simulink model "smartHome6"  (Simulink 9.1)
settings: Solver=VariableStepAuto  StartTime=0.0  StopTime=100  RelTol=1e-3
libraries: commrandsrc3 x21, simulink x8
settings Model: Creator=afarooq  LastModifiedBy=afarooq
settings DataIOCC: SaveFormat=Dataset
settings OptimizationCC: LifeSpan=auto
settings DebuggingCC: UnderspecifiedInitializationDetection=Simplified  MergeDetectMultiDrivingBlocksExec=error  SFUnexpectedBacktrackingDiag=error  SFNoUnconditionalDefaultTransitionDiag=error  SFExecutionAtInitializationDiag=warning
settings HardwareCC: ProdBitPerPointer=64  ProdBitPerSizeT=64  ProdBitPerPtrDiffT=64  ProdLargestAtomicFloat=Float  ProdIntDivRoundTo=Zero  ProdEndianess=LittleEndian  ProdWordSize=64  ProdHWDeviceType=Intel->x86-64 (Windows64)
settings ModelReferenceCC: PropagateSignalLabelsOutOfModel=on
settings CodeAppCC: StateflowObjectComments=off
settings GRTTargetCC: TargetLangStandard=C99 (ISO)  CombineOutputUpdateFcns=on  GRTInterface=off
settings ConfigComp: CovMetricSettings=dwe  CovHtmlReporting=off  CovSaveCumulativeToWorkspaceVar=off  CovSaveSingleToWorkspaceVar=off  CovExternalEMLEnable=on

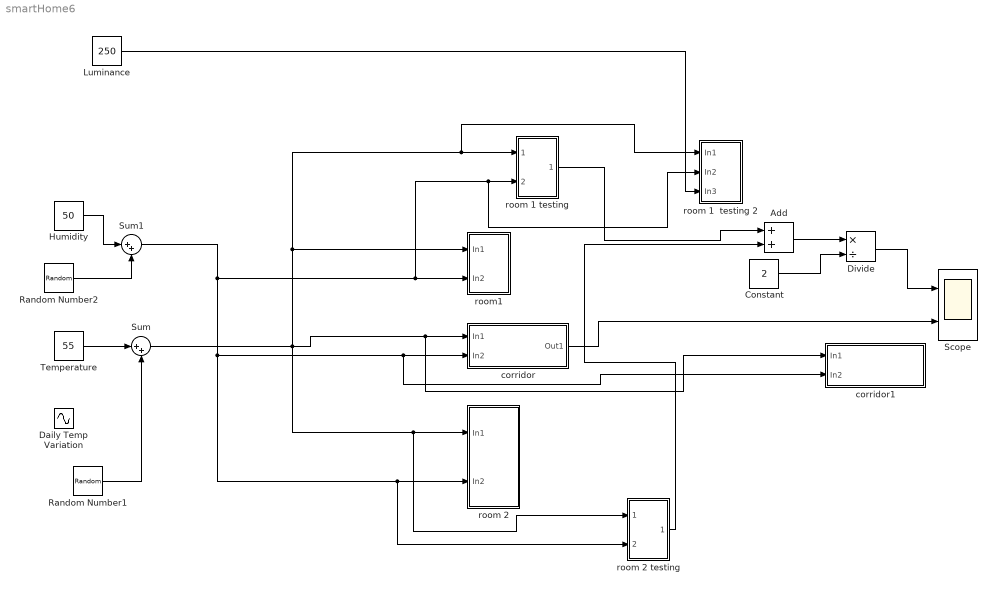
== system smartHome6 ==
  Add : Sum
  Constant : Constant  Value=2
  Daily Temp Variation : Sin  Amplitude=10  Frequency=2*pi/24  SampleTime=0
  Divide : Product  Inputs=*/
  Humidity : Constant  Value=50
  Luminance : Constant  Value=250
  Random Number1 : RandomNumber  Mean=10  Variance=15  SampleTime=1.0
  Random Number2 : RandomNumber  Mean=10  Variance=15  SampleTime=1.0
  Scope : Scope  NumInputPorts=2
  Sum : Sum  Inputs=|++
  Sum1 : Sum  Inputs=|++
  Temperature : Constant  Value=55
  corridor : Subsystem
  corridor1 : Subsystem
  room 1  testing 2 : Subsystem
  "room 1 testing " : Subsystem
  room 2 : Subsystem
  "room 2 testing " : Subsystem
  room1 : Subsystem
  wires:
  Temperature/1 -> Sum/1
  Humidity/1 -> Sum1/1
  Random Number2/1 -> Sum1/2
  Random Number1/1 -> Sum/2
  corridor/1(Out1) -> Scope/2
  Sum1/1 -> "room 2 testing "/2(In2), room 2/2(In2), corridor1/2(In2), corridor/2(In2), room 1  testing 2/2(In2), "room 1 testing "/2(In2), room1/2(In2)
  Sum/1 -> corridor1/1(In1), corridor/1(In1), "room 2 testing "/1(In1), room 2/1(In1), room 1  testing 2/1(In1), "room 1 testing "/1(In1), room1/1(In1)
  "room 1 testing "/1(Out1) -> Add/1
  "room 2 testing "/1(Out1) -> Add/2
  Add/1 -> Divide/1
  Constant/1 -> Divide/2
  Divide/1 -> Scope/1
  Luminance/1 -> room 1  testing 2/3(In3)

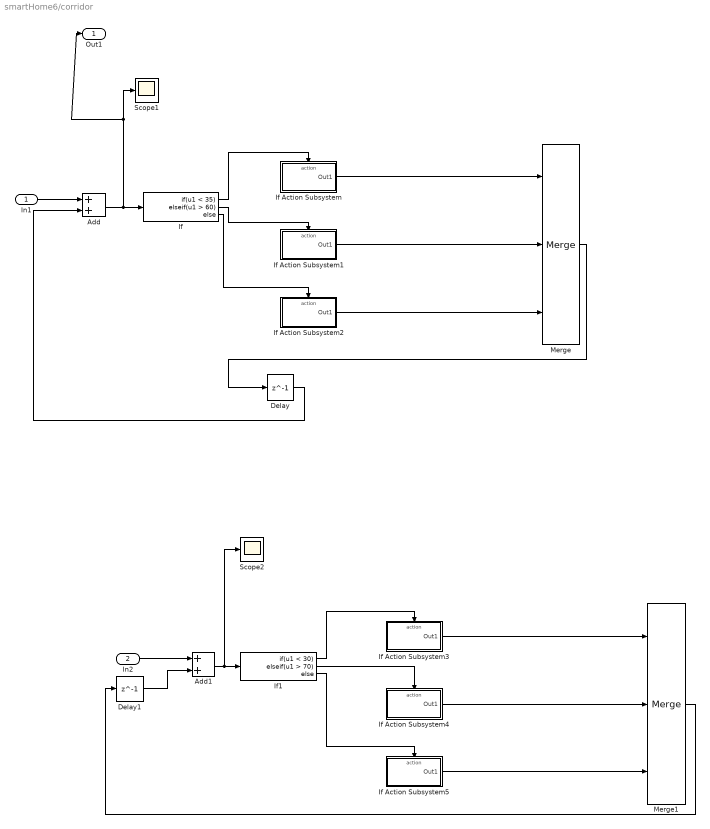
== system smartHome6/corridor ==
  In1 : Inport
  In2 : Inport  Port=2
  Add : Sum
  Add1 : Sum
  Delay : Delay  DelayLength=1  InitialCondition=0
  Delay1 : Delay  DelayLength=1  InitialCondition=0
  If : If  IfExpression=u1 < 35  ElseIfExpressions=u1 > 60
  If Action Subsystem : Subsystem  TreatAsAtomicUnit=on
  If Action Subsystem1 : Subsystem  TreatAsAtomicUnit=on
  If Action Subsystem2 : Subsystem  TreatAsAtomicUnit=on
  If Action Subsystem3 : Subsystem  TreatAsAtomicUnit=on
  If Action Subsystem4 : Subsystem  TreatAsAtomicUnit=on
  If Action Subsystem5 : Subsystem  TreatAsAtomicUnit=on
  If1 : If  IfExpression=u1 < 30  ElseIfExpressions=u1 > 70
  Merge : Merge  Inputs=3
  Merge1 : Merge  Inputs=3
  Scope1 : Scope
  Scope2 : Scope
  Out1 : Outport
  wires:
  If Action Subsystem1/1(Out1) -> Merge/2
  Merge/1 -> Delay/1
  Add/1 -> Out1/1, Scope1/1, If/1
  If/1 -> If Action Subsystem/Action
  If/2 -> If Action Subsystem1/Action
  If/3 -> If Action Subsystem2/Action
  In1/1 -> Add/1
  If Action Subsystem2/1(Out1) -> Merge/3
  If Action Subsystem/1(Out1) -> Merge/1
  Delay/1 -> Add/2
  In2/1 -> Add1/1
  Delay1/1 -> Add1/2
  Add1/1 -> Scope2/1, If1/1
  If1/2 -> If Action Subsystem4/Action
  If1/3 -> If Action Subsystem5/Action
  If Action Subsystem3/1(Out1) -> Merge1/1
  If1/1 -> If Action Subsystem3/Action
  If Action Subsystem4/1(Out1) -> Merge1/2
  Merge1/1 -> Delay1/1
  If Action Subsystem5/1(Out1) -> Merge1/3

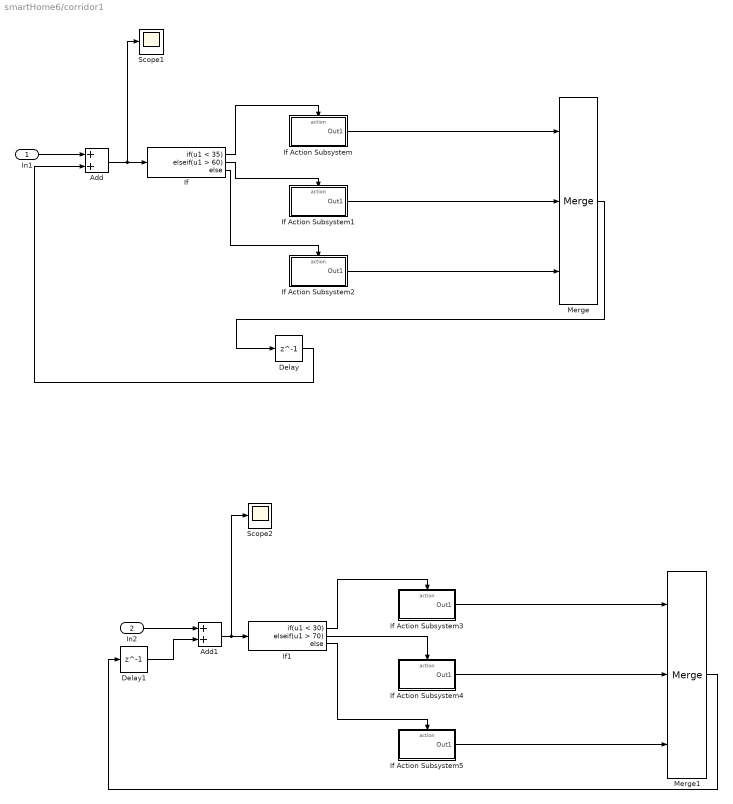
== system smartHome6/corridor1 ==
  In1 : Inport
  In2 : Inport  Port=2
  Add : Sum
  Add1 : Sum
  Delay : Delay  DelayLength=1  InitialCondition=0
  Delay1 : Delay  DelayLength=1  InitialCondition=0
  If : If  IfExpression=u1 < 35  ElseIfExpressions=u1 > 60
  If Action Subsystem : Subsystem  TreatAsAtomicUnit=on
  If Action Subsystem1 : Subsystem  TreatAsAtomicUnit=on
  If Action Subsystem2 : Subsystem  TreatAsAtomicUnit=on
  If Action Subsystem3 : Subsystem  TreatAsAtomicUnit=on
  If Action Subsystem4 : Subsystem  TreatAsAtomicUnit=on
  If Action Subsystem5 : Subsystem  TreatAsAtomicUnit=on
  If1 : If  IfExpression=u1 < 30  ElseIfExpressions=u1 > 70
  Merge : Merge  Inputs=3
  Merge1 : Merge  Inputs=3
  Scope1 : Scope
  Scope2 : Scope
  wires:
  If Action Subsystem1/1(Out1) -> Merge/2
  Merge/1 -> Delay/1
  Add/1 -> Scope1/1, If/1
  If/1 -> If Action Subsystem/Action
  If/2 -> If Action Subsystem1/Action
  If/3 -> If Action Subsystem2/Action
  In1/1 -> Add/1
  If Action Subsystem2/1(Out1) -> Merge/3
  If Action Subsystem/1(Out1) -> Merge/1
  Delay/1 -> Add/2
  In2/1 -> Add1/1
  Delay1/1 -> Add1/2
  Add1/1 -> Scope2/1, If1/1
  If1/2 -> If Action Subsystem4/Action
  If1/3 -> If Action Subsystem5/Action
  If Action Subsystem3/1(Out1) -> Merge1/1
  If1/1 -> If Action Subsystem3/Action
  If Action Subsystem4/1(Out1) -> Merge1/2
  Merge1/1 -> Delay1/1
  If Action Subsystem5/1(Out1) -> Merge1/3

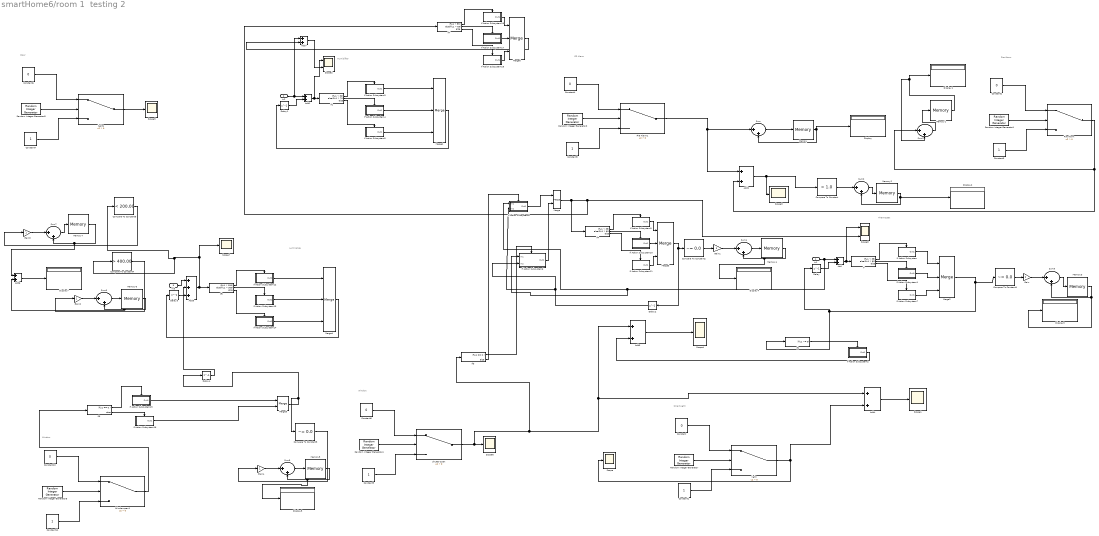
== system smartHome6/room 1  testing 2 ==
  note: Smart Light
  note: Humidifier
  note: Thermostat
  note: Fire Alarm
  note: CO Alarm
  note: Door
  note: Window
  note: Luminance
  note: Window
  In1 : Inport
  In2 : Inport  Port=2
  In3 : Inport  Port=3
  Add{,1..4,6..7} (7 alike) : Sum
  Add5 : Sum  Inputs=+++
  Compare To Constant : simulink/Logic and Bit Operations/Compare To Constant  relop=>  const=1.0  OutDataTypeStr=uint8
  Compare To Constant1 : simulink/Logic and Bit Operations/Compare To Constant  relop=~=  const=0.0  OutDataTypeStr=uint8
  Compare To Constant2 : simulink/Logic and Bit Operations/Compare To Constant  relop=~=  const=0.0  OutDataTypeStr=uint8
  Compare To Constant3 : simulink/Logic and Bit Operations/Compare To Constant  relop=~=  const=0.0  OutDataTypeStr=uint8
  Compare To Constant4 : simulink/Logic and Bit Operations/Compare To Constant  relop=>  const=400.00  OutDataTypeStr=uint8
  Compare To Constant5 : simulink/Logic and Bit Operations/Compare To Constant  relop=<  const=200.00  OutDataTypeStr=uint8
  Constant{,2,4,6,8,10} (6 alike) : Constant  Value=0
  Constant{1,3,5,7,9,11} (6 alike) : Constant
  Delay{,1..4} (5 alike) : Delay  DelayLength=1  InitialCondition=0
  Display{,1..5,7} (7 alike) : Display
  Fire Alarm : Switch  Criteria=u2 > Threshold
  Fire Alarm1 : Switch  Criteria=u2 > Threshold
  Gain{,1..4} (5 alike) : Gain
  If : If  IfExpression=u1 < 35  ElseIfExpressions=u1 > 60
  If Action Subsystem : Subsystem  TreatAsAtomicUnit=on
  If Action Subsystem1 : Subsystem  TreatAsAtomicUnit=on
  If Action Subsystem10 : Subsystem  TreatAsAtomicUnit=on
  If Action Subsystem11 : Subsystem  TreatAsAtomicUnit=on
  If Action Subsystem12 : Subsystem  TreatAsAtomicUnit=on
  If Action Subsystem13 : Subsystem  TreatAsAtomicUnit=on
  If Action Subsystem14 : Subsystem  TreatAsAtomicUnit=on
  If Action Subsystem15 : Subsystem  TreatAsAtomicUnit=on
  If Action Subsystem16 : Subsystem  TreatAsAtomicUnit=on
  If Action Subsystem17 : Subsystem  TreatAsAtomicUnit=on
  If Action Subsystem18 : Subsystem  TreatAsAtomicUnit=on
  If Action Subsystem19 : Subsystem  TreatAsAtomicUnit=on
  If Action Subsystem2 : Subsystem  TreatAsAtomicUnit=on
  If Action Subsystem3 : Subsystem  TreatAsAtomicUnit=on
  If Action Subsystem4 : Subsystem  TreatAsAtomicUnit=on
  If Action Subsystem5 : Subsystem  TreatAsAtomicUnit=on
  If Action Subsystem6 : Subsystem  TreatAsAtomicUnit=on
  If Action Subsystem7 : Subsystem  TreatAsAtomicUnit=on
  If Action Subsystem8 : Subsystem  TreatAsAtomicUnit=on
  If Action Subsystem9 : Subsystem  TreatAsAtomicUnit=on
  If1 : If  IfExpression=u1 < 30  ElseIfExpressions=u1 > 70
  If2 : If  IfExpression=u1 ~= 0  ShowElse=off
  If3 : If  IfExpression=u1 == 0
  If4 : If  IfExpression=u1 < 35  ElseIfExpressions=u1 > 60
  If5 : If  IfExpression=u1 < 150  ElseIfExpressions=u1 > 300
  If6 : If  IfExpression=u1 == 0
  If7 : If  IfExpression=u1 < 55  ElseIfExpressions=u1 > 65
  Memory{,1..7} (8 alike) : Memory
  Merge : Merge
  Merge{1..4,6} (5 alike) : Merge  Inputs=3
  Merge5 : Merge
  Random Integer Generator : commrandsrc3/Random Integer Generator  SetSize=3  SeedSource=Auto  Seed=0  SampleTime=1  SamplesPerFrame=1  OutputDataType=double  SimulateUsing=Interpreted execution
  Random Integer Generator1 : commrandsrc3/Random Integer Generator  SetSize=8  SeedSource=Auto  Seed=0  SampleTime=1  SamplesPerFrame=1  OutputDataType=double  SimulateUsing=Interpreted execution
  Random Integer Generator2 : commrandsrc3/Random Integer Generator  SetSize=30  SeedSource=Auto  Seed=0  SampleTime=1  SamplesPerFrame=1  OutputDataType=double  SimulateUsing=Interpreted execution
  Random Integer Generator3 : commrandsrc3/Random Integer Generator  SetSize=10  SeedSource=Auto  Seed=0  SampleTime=1  SamplesPerFrame=1  OutputDataType=double  SimulateUsing=Interpreted execution
  Random Integer Generator4 : commrandsrc3/Random Integer Generator  SetSize=10  SeedSource=Auto  Seed=0  SampleTime=1  SamplesPerFrame=1  OutputDataType=double  SimulateUsing=Interpreted execution
  Random Integer Generator5 : commrandsrc3/Random Integer Generator  SetSize=15  SeedSource=Auto  Seed=0  SampleTime=1  SamplesPerFrame=1  OutputDataType=double  SimulateUsing=Interpreted execution
  Scope{,1,3..7} (7 alike) : Scope
  Scope2 : Scope  NumInputPorts=2
  Scope8 : Scope  NumInputPorts=2
  Sum{,1..7} (8 alike) : Sum  Inputs=|++
  blinder open1 : Switch  Criteria=u2 > Threshold
  light : Switch  Criteria=u2 > Threshold
  light1 : Switch  Criteria=u2 > Threshold
  shutter open : Switch  Criteria=u2 > Threshold
  wires:
  If/2 -> If Action Subsystem1/Action
  If/1 -> If Action Subsystem/Action
  In1/1 -> If Action Subsystem8/1(In1), If Action Subsystem6/1(In1), Add/1
  Add/1 -> Scope8/1, If/1
  Delay/1 -> Add/2
  If Action Subsystem4/1(Out1) -> Merge1/2
  If Action Subsystem5/1(Out1) -> Merge1/3
  If Action Subsystem3/1(Out1) -> Merge1/1
  Merge1/1 -> Delay1/1
  If1/3 -> If Action Subsystem5/Action
  If1/1 -> If Action Subsystem3/Action
  If1/2 -> If Action Subsystem4/Action
  Add1/1 -> Scope2/1, If1/1
  Delay1/1 -> Add1/2
  Random Integer Generator/1 -> light/2
  Constant/1 -> light/1
  Constant1/1 -> light/3
  light/1 -> Add4/2, Scope/1
  Constant2/1 -> Fire Alarm/1
  Constant3/1 -> Fire Alarm/3
  Random Integer Generator1/1 -> Fire Alarm/2
  Random Integer Generator2/1 -> Fire Alarm1/2
  Constant5/1 -> Fire Alarm1/3
  Fire Alarm1/1 -> Add2/1, Sum/1
  Constant4/1 -> Fire Alarm1/1
  Constant6/1 -> light1/1
  Constant7/1 -> light1/3
  Random Integer Generator3/1 -> light1/2
  light1/1 -> Scope5/1
  Random Integer Generator4/1 -> shutter open/2
  shutter open/1 -> If3/1, Add4/1, Add3/1, Scope6/1
  Constant8/1 -> shutter open/1
  Constant9/1 -> shutter open/3
  If Action Subsystem/1(Out1) -> Merge2/1
  If Action Subsystem1/1(Out1) -> Merge2/2
  Merge2/1 -> Compare To Constant1/1, Delay/1, If2/1
  If2/1 -> If Action Subsystem2/Action
  If Action Subsystem2/1(Out1) -> Add3/2
  Add3/1 -> Scope4/1
  Add2/1 -> Compare To Constant/1, Scope3/1
  If/3 -> If Action Subsystem7/Action
  If Action Subsystem7/1(Out1) -> Merge2/3
  Delay2/1 -> If Action Subsystem8/2(In2), If Action Subsystem6/2(In2)
  If Action Subsystem6/1(Out1) -> Merge/2
  Add4/1 -> Scope1/1
  Sum/1 -> Memory/1
  Memory/1 -> Display/1, Sum/2
  Memory1/1 -> Sum1/2, Display1/1
  Sum1/1 -> Memory1/1
  Fire Alarm/1 -> Sum1/1, Add2/2
  Memory2/1 -> Display2/1, Sum2/2
  Sum2/1 -> Memory2/1
  Compare To Constant/1 -> Sum2/1
  If Action Subsystem8/1(Out1) -> Merge/1
  If Action Subsystem11/1(Out1) -> Merge3/3
  If4/1 -> If Action Subsystem9/Action
  If Action Subsystem9/1(Out1) -> Merge3/1
  If4/3 -> If Action Subsystem11/Action
  If Action Subsystem10/1(Out1) -> Merge3/2
  If4/2 -> If Action Subsystem10/Action
  Merge3/1 -> Delay2/1, Compare To Constant2/1
  Sum3/1 -> Memory3/1
  Memory3/1 -> Display3/1, Sum3/2
  Sum4/1 -> Memory4/1
  Memory4/1 -> Sum4/2, Display4/1
  Compare To Constant1/1 -> Gain/1
  Gain/1 -> Sum3/1
  Compare To Constant2/1 -> Gain1/1
  Gain1/1 -> Sum4/1
  Delay3/1 -> Add5/3
  If Action Subsystem12/1(Out1) -> Merge4/1
  If5/1 -> If Action Subsystem12/Action
  Merge4/1 -> Delay3/1
  If Action Subsystem13/1(Out1) -> Merge4/2
  If5/3 -> If Action Subsystem14/Action
  If5/2 -> If Action Subsystem13/Action
  In3/1 -> Add5/1
  If Action Subsystem14/1(Out1) -> Merge4/3
  If3/2 -> If Action Subsystem8/Action
  If3/1 -> If Action Subsystem6/Action
  Merge5/1 -> Compare To Constant3/1, Delay4/1
  Delay4/1 -> Add5/2
  Memory5/1 -> Sum5/2, Display5/1
  Gain4/1 -> Sum5/1
  Sum5/1 -> Memory5/1
  Constant11/1 -> blinder open1/3
  Random Integer Generator5/1 -> blinder open1/2
  Constant10/1 -> blinder open1/1
  blinder open1/1 -> If6/1
  If6/1 -> If Action Subsystem15/Action
  If Action Subsystem15/1(Out1) -> Merge5/1
  If6/2 -> If Action Subsystem16/Action
  If Action Subsystem16/1(Out1) -> Merge5/2
  Compare To Constant3/1 -> Gain4/1
  Gain2/1 -> Sum6/1
  Compare To Constant4/1 -> Gain2/1
  Memory6/1 -> Add6/2, Sum6/2
  Sum6/1 -> Memory6/1
  Compare To Constant5/1 -> Gain3/1
  Sum7/1 -> Memory7/1
  Memory7/1 -> Add6/1, Sum7/2
  Gain3/1 -> Sum7/1
  Add5/1 -> Compare To Constant5/1, Compare To Constant4/1, Scope7/1, If5/1
  Add6/1 -> Display7/1
  Add7/1 -> Scope2/2
  If Action Subsystem17/1(Out1) -> Merge6/2
  Merge6/1 -> Add7/2
  If7/2 -> If Action Subsystem17/Action
  If7/3 -> If Action Subsystem18/Action
  Merge/1 -> If4/1, If7/1, Scope8/2
  If7/1 -> If Action Subsystem19/Action
  If Action Subsystem18/1(Out1) -> Merge6/3
  If Action Subsystem19/1(Out1) -> Merge6/1
  In2/1 -> Add7/1, Add1/1

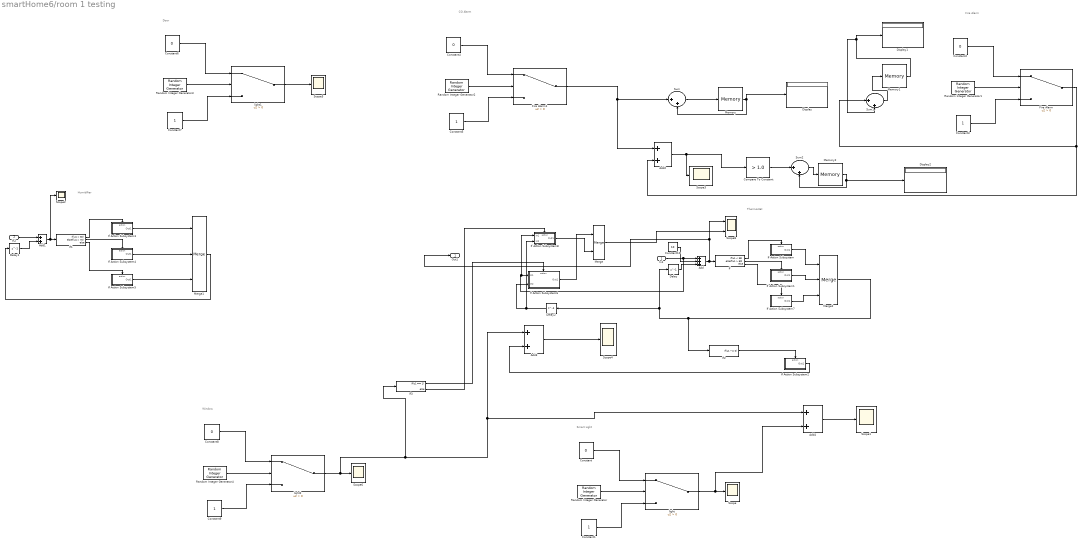
== system smartHome6/room 1 testing  ==
  note: Smart Light
  note: Humidifier
  note: Thermostat
  note: Fire Alarm
  note: CO Alarm
  note: Door
  note: Window
  In1 : Inport
  In2 : Inport  Port=2
  Add : Sum  Inputs=+++
  Add{1..4} (4 alike) : Sum
  Compare To Constant : simulink/Logic and Bit Operations/Compare To Constant  relop=>  const=1.0  OutDataTypeStr=uint8
  Constant{,2,4,6,8} (5 alike) : Constant  Value=0
  Constant{1,3,5,7,9} (5 alike) : Constant
  Constant10 : Constant  Value=10
  Delay : Delay  DelayLength=1  InitialCondition=0
  Delay1 : Delay  DelayLength=1  InitialCondition=0
  Delay2 : Delay  DelayLength=1  InitialCondition=0
  Display : Display
  Display1 : Display
  Display2 : Display
  Fire Alarm : Switch  Criteria=u2 > Threshold
  Fire Alarm1 : Switch  Criteria=u2 > Threshold
  If : If  IfExpression=u1 < 35  ElseIfExpressions=u1 > 60
  If Action Subsystem : Subsystem  TreatAsAtomicUnit=on
  If Action Subsystem1 : Subsystem  TreatAsAtomicUnit=on
  If Action Subsystem2 : Subsystem  TreatAsAtomicUnit=on
  If Action Subsystem3 : Subsystem  TreatAsAtomicUnit=on
  If Action Subsystem4 : Subsystem  TreatAsAtomicUnit=on
  If Action Subsystem5 : Subsystem  TreatAsAtomicUnit=on
  If Action Subsystem6 : Subsystem  TreatAsAtomicUnit=on
  If Action Subsystem7 : Subsystem  TreatAsAtomicUnit=on
  If Action Subsystem8 : Subsystem  TreatAsAtomicUnit=on
  If1 : If  IfExpression=u1 < 30  ElseIfExpressions=u1 > 70
  If2 : If  IfExpression=u1 ~= 0  ShowElse=off
  If3 : If  IfExpression=u1 == 1
  Memory : Memory
  Memory1 : Memory
  Memory2 : Memory
  Merge : Merge
  Merge1 : Merge  Inputs=3
  Merge2 : Merge  Inputs=3
  Random Integer Generator : commrandsrc3/Random Integer Generator  SetSize=3  SeedSource=Auto  Seed=0  SampleTime=1  SamplesPerFrame=1  OutputDataType=double  SimulateUsing=Interpreted execution
  Random Integer Generator1 : commrandsrc3/Random Integer Generator  SetSize=8  SeedSource=Auto  Seed=0  SampleTime=1  SamplesPerFrame=1  OutputDataType=double  SimulateUsing=Interpreted execution
  Random Integer Generator2 : commrandsrc3/Random Integer Generator  SetSize=30  SeedSource=Auto  Seed=0  SampleTime=1  SamplesPerFrame=1  OutputDataType=double  SimulateUsing=Interpreted execution
  Random Integer Generator3 : commrandsrc3/Random Integer Generator  SetSize=10  SeedSource=Auto  Seed=0  SampleTime=1  SamplesPerFrame=1  OutputDataType=double  SimulateUsing=Interpreted execution
  Random Integer Generator4 : commrandsrc3/Random Integer Generator  SetSize=10  SeedSource=Auto  Seed=0  SampleTime=1  SamplesPerFrame=1  OutputDataType=double  SimulateUsing=Interpreted execution
  Scope{,1..6} (7 alike) : Scope
  Scope8 : Scope  NumInputPorts=2
  Sum : Sum  Inputs=|++
  Sum1 : Sum  Inputs=|++
  Sum2 : Sum  Inputs=|++
  light : Switch  Criteria=u2 > Threshold
  light1 : Switch  Criteria=u2 > Threshold
  light2 : Switch  Criteria=u2 > Threshold
  Out1 : Outport
  wires:
  If/2 -> If Action Subsystem1/Action
  If/1 -> If Action Subsystem/Action
  In1/1 -> If Action Subsystem8/1(In1), If Action Subsystem6/1(In1), Add/1
  Add/1 -> Out1/1, Scope8/1, If/1
  Delay/1 -> Add/3
  If Action Subsystem4/1(Out1) -> Merge1/2
  If Action Subsystem5/1(Out1) -> Merge1/3
  If Action Subsystem3/1(Out1) -> Merge1/1
  Merge1/1 -> Delay1/1
  In2/1 -> Add1/1
  If1/3 -> If Action Subsystem5/Action
  If1/1 -> If Action Subsystem3/Action
  If1/2 -> If Action Subsystem4/Action
  Add1/1 -> Scope2/1, If1/1
  Delay1/1 -> Add1/2
  Random Integer Generator/1 -> light/2
  Constant/1 -> light/1
  Constant1/1 -> light/3
  light/1 -> Add4/2, Scope/1
  Constant2/1 -> Fire Alarm/1
  Constant3/1 -> Fire Alarm/3
  Random Integer Generator1/1 -> Fire Alarm/2
  Random Integer Generator2/1 -> Fire Alarm1/2
  Constant5/1 -> Fire Alarm1/3
  Fire Alarm1/1 -> Add2/1, Sum/1
  Constant4/1 -> Fire Alarm1/1
  Constant6/1 -> light1/1
  Constant7/1 -> light1/3
  Random Integer Generator3/1 -> light1/2
  light1/1 -> Scope5/1
  Random Integer Generator4/1 -> light2/2
  light2/1 -> If3/1, Add4/1, Add3/1, Scope6/1
  Constant8/1 -> light2/1
  Constant9/1 -> light2/3
  If Action Subsystem/1(Out1) -> Merge2/1
  If Action Subsystem1/1(Out1) -> Merge2/2
  Merge2/1 -> If2/1, Delay/1, Delay2/1
  If2/1 -> If Action Subsystem2/Action
  If Action Subsystem2/1(Out1) -> Add3/2
  Add3/1 -> Scope4/1
  Add2/1 -> Compare To Constant/1, Scope3/1
  If/3 -> If Action Subsystem7/Action
  If Action Subsystem7/1(Out1) -> Merge2/3
  If3/1 -> If Action Subsystem6/Action
  Delay2/1 -> If Action Subsystem8/2(In2), If Action Subsystem6/2(In2)
  If3/2 -> If Action Subsystem8/Action
  If Action Subsystem6/1(Out1) -> Merge/1
  Merge/1 -> Scope8/2
  If Action Subsystem8/1(Out1) -> Merge/2
  Add4/1 -> Scope1/1
  Sum/1 -> Memory/1
  Memory/1 -> Display/1, Sum/2
  Memory1/1 -> Sum1/2, Display1/1
  Sum1/1 -> Memory1/1
  Fire Alarm/1 -> Sum1/1, Add2/2
  Memory2/1 -> Display2/1, Sum2/2
  Sum2/1 -> Memory2/1
  Compare To Constant/1 -> Sum2/1
  Constant10/1 -> Add/2

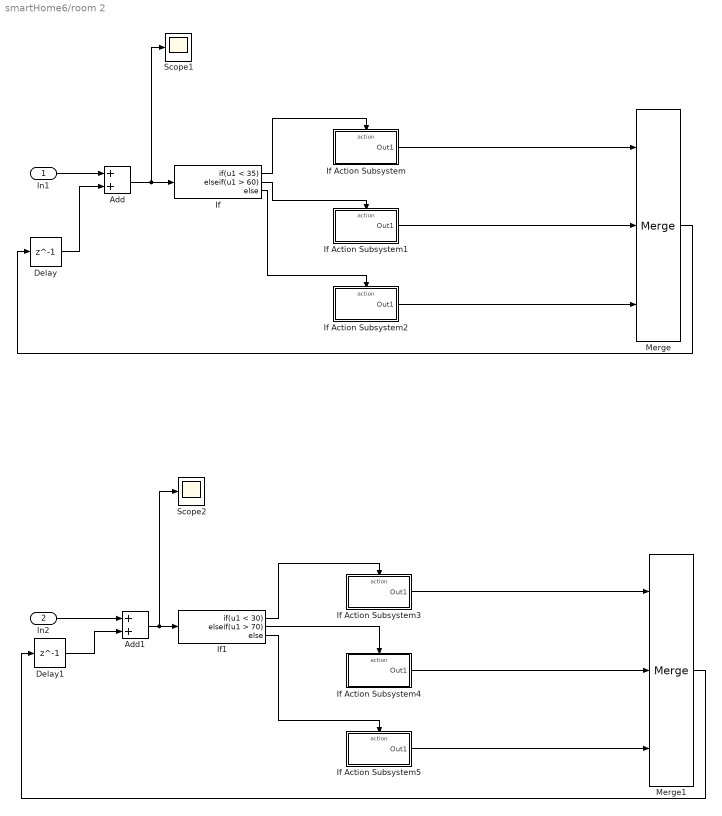
== system smartHome6/room 2 ==
  In1 : Inport
  In2 : Inport  Port=2
  Add : Sum
  Add1 : Sum
  Delay : Delay  DelayLength=1  InitialCondition=0
  Delay1 : Delay  DelayLength=1  InitialCondition=0
  If : If  IfExpression=u1 < 35  ElseIfExpressions=u1 > 60
  If Action Subsystem : Subsystem  TreatAsAtomicUnit=on
  If Action Subsystem1 : Subsystem  TreatAsAtomicUnit=on
  If Action Subsystem2 : Subsystem  TreatAsAtomicUnit=on
  If Action Subsystem3 : Subsystem  TreatAsAtomicUnit=on
  If Action Subsystem4 : Subsystem  TreatAsAtomicUnit=on
  If Action Subsystem5 : Subsystem  TreatAsAtomicUnit=on
  If1 : If  IfExpression=u1 < 30  ElseIfExpressions=u1 > 70
  Merge : Merge  Inputs=3
  Merge1 : Merge  Inputs=3
  Scope1 : Scope
  Scope2 : Scope
  wires:
  If Action Subsystem1/1(Out1) -> Merge/2
  Merge/1 -> Delay/1
  Add/1 -> Scope1/1, If/1
  If/1 -> If Action Subsystem/Action
  If/2 -> If Action Subsystem1/Action
  If/3 -> If Action Subsystem2/Action
  In1/1 -> Add/1
  If Action Subsystem2/1(Out1) -> Merge/3
  If Action Subsystem/1(Out1) -> Merge/1
  Delay/1 -> Add/2
  Merge1/1 -> Delay1/1
  If1/1 -> If Action Subsystem3/Action
  If Action Subsystem4/1(Out1) -> Merge1/2
  If1/3 -> If Action Subsystem5/Action
  Add1/1 -> Scope2/1, If1/1
  If1/2 -> If Action Subsystem4/Action
  If Action Subsystem3/1(Out1) -> Merge1/1
  Delay1/1 -> Add1/2
  In2/1 -> Add1/1
  If Action Subsystem5/1(Out1) -> Merge1/3

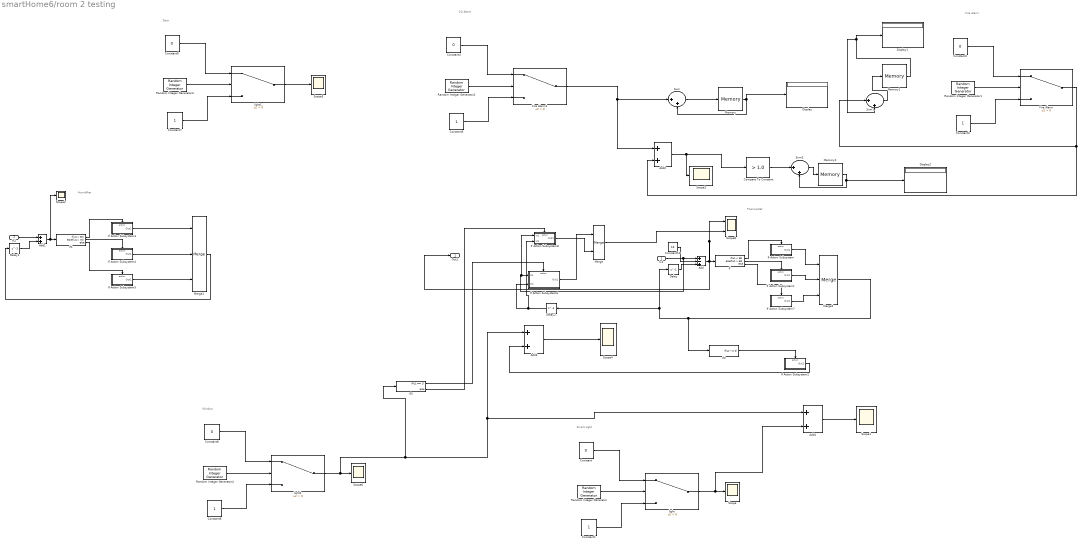
== system smartHome6/room 2 testing  ==
  note: Smart Light
  note: Humidifier
  note: Thermostat
  note: Fire Alarm
  note: CO Alarm
  note: Door
  note: Window
  In1 : Inport
  In2 : Inport  Port=2
  Add : Sum  Inputs=+-+
  Add{1..4} (4 alike) : Sum
  Compare To Constant : simulink/Logic and Bit Operations/Compare To Constant  relop=>  const=1.0  OutDataTypeStr=uint8
  Constant{,2,4,6,8} (5 alike) : Constant  Value=0
  Constant{1,3,5,7,9} (5 alike) : Constant
  Constant10 : Constant  Value=10
  Delay : Delay  DelayLength=1  InitialCondition=0
  Delay1 : Delay  DelayLength=1  InitialCondition=0
  Delay2 : Delay  DelayLength=1  InitialCondition=0
  Display : Display
  Display1 : Display
  Display2 : Display
  Fire Alarm : Switch  Criteria=u2 > Threshold
  Fire Alarm1 : Switch  Criteria=u2 > Threshold
  If : If  IfExpression=u1 < 35  ElseIfExpressions=u1 > 60
  If Action Subsystem : Subsystem  TreatAsAtomicUnit=on
  If Action Subsystem1 : Subsystem  TreatAsAtomicUnit=on
  If Action Subsystem2 : Subsystem  TreatAsAtomicUnit=on
  If Action Subsystem3 : Subsystem  TreatAsAtomicUnit=on
  If Action Subsystem4 : Subsystem  TreatAsAtomicUnit=on
  If Action Subsystem5 : Subsystem  TreatAsAtomicUnit=on
  If Action Subsystem6 : Subsystem  TreatAsAtomicUnit=on
  If Action Subsystem7 : Subsystem  TreatAsAtomicUnit=on
  If Action Subsystem8 : Subsystem  TreatAsAtomicUnit=on
  If1 : If  IfExpression=u1 < 30  ElseIfExpressions=u1 > 70
  If2 : If  IfExpression=u1 ~= 0  ShowElse=off
  If3 : If  IfExpression=u1 == 1
  Memory : Memory
  Memory1 : Memory
  Memory2 : Memory
  Merge : Merge
  Merge1 : Merge  Inputs=3
  Merge2 : Merge  Inputs=3
  Random Integer Generator : commrandsrc3/Random Integer Generator  SetSize=3  SeedSource=Auto  Seed=0  SampleTime=1  SamplesPerFrame=1  OutputDataType=double  SimulateUsing=Interpreted execution
  Random Integer Generator1 : commrandsrc3/Random Integer Generator  SetSize=8  SeedSource=Auto  Seed=0  SampleTime=1  SamplesPerFrame=1  OutputDataType=double  SimulateUsing=Interpreted execution
  Random Integer Generator2 : commrandsrc3/Random Integer Generator  SetSize=30  SeedSource=Auto  Seed=0  SampleTime=1  SamplesPerFrame=1  OutputDataType=double  SimulateUsing=Interpreted execution
  Random Integer Generator3 : commrandsrc3/Random Integer Generator  SetSize=10  SeedSource=Auto  Seed=0  SampleTime=1  SamplesPerFrame=1  OutputDataType=double  SimulateUsing=Interpreted execution
  Random Integer Generator4 : commrandsrc3/Random Integer Generator  SetSize=10  SeedSource=Auto  Seed=0  SampleTime=1  SamplesPerFrame=1  OutputDataType=double  SimulateUsing=Interpreted execution
  Scope{,1..6} (7 alike) : Scope
  Scope8 : Scope  NumInputPorts=2
  Sum : Sum  Inputs=|++
  Sum1 : Sum  Inputs=|++
  Sum2 : Sum  Inputs=|++
  light : Switch  Criteria=u2 > Threshold
  light1 : Switch  Criteria=u2 > Threshold
  light2 : Switch  Criteria=u2 > Threshold
  Out1 : Outport
  wires:
  If/2 -> If Action Subsystem1/Action
  If/1 -> If Action Subsystem/Action
  In1/1 -> If Action Subsystem8/1(In1), If Action Subsystem6/1(In1), Add/1
  Add/1 -> Out1/1, Scope8/1, If/1
  Delay/1 -> Add/3
  If Action Subsystem4/1(Out1) -> Merge1/2
  If Action Subsystem5/1(Out1) -> Merge1/3
  If Action Subsystem3/1(Out1) -> Merge1/1
  Merge1/1 -> Delay1/1
  In2/1 -> Add1/1
  If1/3 -> If Action Subsystem5/Action
  If1/1 -> If Action Subsystem3/Action
  If1/2 -> If Action Subsystem4/Action
  Add1/1 -> Scope2/1, If1/1
  Delay1/1 -> Add1/2
  Random Integer Generator/1 -> light/2
  Constant/1 -> light/1
  Constant1/1 -> light/3
  light/1 -> Add4/2, Scope/1
  Constant2/1 -> Fire Alarm/1
  Constant3/1 -> Fire Alarm/3
  Random Integer Generator1/1 -> Fire Alarm/2
  Random Integer Generator2/1 -> Fire Alarm1/2
  Constant5/1 -> Fire Alarm1/3
  Fire Alarm1/1 -> Add2/1, Sum/1
  Constant4/1 -> Fire Alarm1/1
  Constant6/1 -> light1/1
  Constant7/1 -> light1/3
  Random Integer Generator3/1 -> light1/2
  light1/1 -> Scope5/1
  Random Integer Generator4/1 -> light2/2
  light2/1 -> If3/1, Add4/1, Add3/1, Scope6/1
  Constant8/1 -> light2/1
  Constant9/1 -> light2/3
  If Action Subsystem/1(Out1) -> Merge2/1
  If Action Subsystem1/1(Out1) -> Merge2/2
  Merge2/1 -> If2/1, Delay/1, Delay2/1
  If2/1 -> If Action Subsystem2/Action
  If Action Subsystem2/1(Out1) -> Add3/2
  Add3/1 -> Scope4/1
  Add2/1 -> Compare To Constant/1, Scope3/1
  If/3 -> If Action Subsystem7/Action
  If Action Subsystem7/1(Out1) -> Merge2/3
  If3/1 -> If Action Subsystem6/Action
  Delay2/1 -> If Action Subsystem8/2(In2), If Action Subsystem6/2(In2)
  If3/2 -> If Action Subsystem8/Action
  If Action Subsystem6/1(Out1) -> Merge/1
  Merge/1 -> Scope8/2
  If Action Subsystem8/1(Out1) -> Merge/2
  Add4/1 -> Scope1/1
  Sum/1 -> Memory/1
  Memory/1 -> Display/1, Sum/2
  Memory1/1 -> Sum1/2, Display1/1
  Sum1/1 -> Memory1/1
  Fire Alarm/1 -> Sum1/1, Add2/2
  Memory2/1 -> Display2/1, Sum2/2
  Sum2/1 -> Memory2/1
  Compare To Constant/1 -> Sum2/1
  Constant10/1 -> Add/2

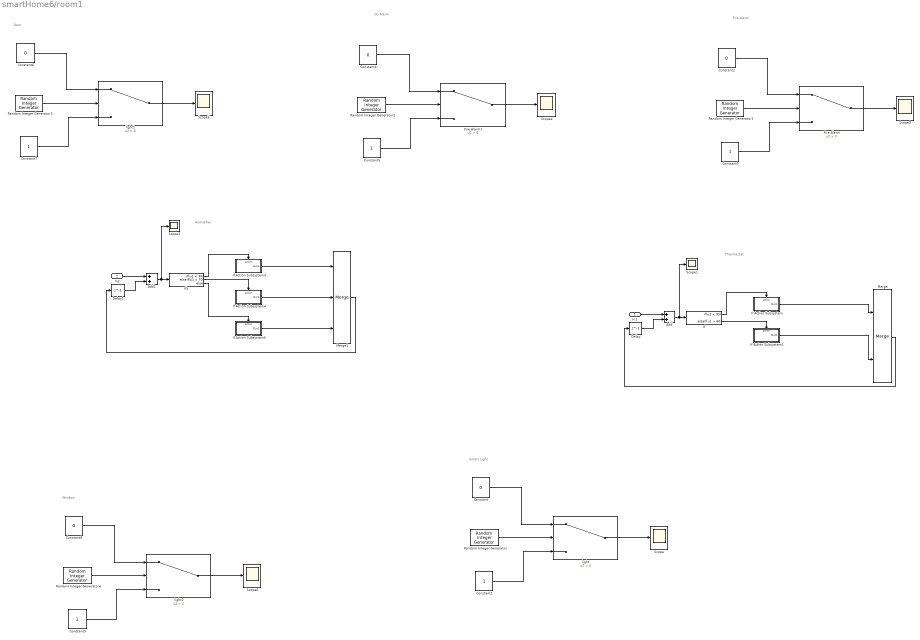
== system smartHome6/room1 ==
  note: Smart Light
  note: Humidifier
  note: Thermostat
  note: Fire Alarm
  note: CO Alarm
  note: Door
  note: Window
  In1 : Inport
  In2 : Inport  Port=2
  Add : Sum
  Add1 : Sum
  Constant{,2,4,6,8} (5 alike) : Constant  Value=0
  Constant{1,3,5,7,9} (5 alike) : Constant
  Delay : Delay  DelayLength=1  InitialCondition=0
  Delay1 : Delay  DelayLength=1  InitialCondition=0
  Fire Alarm : Switch  Criteria=u2 > Threshold
  Fire Alarm1 : Switch  Criteria=u2 > Threshold
  If : If  IfExpression=u1 < 35  ElseIfExpressions=u1 > 60  ShowElse=off
  If Action Subsystem : Subsystem  TreatAsAtomicUnit=on
  If Action Subsystem1 : Subsystem  TreatAsAtomicUnit=on
  If Action Subsystem3 : Subsystem  TreatAsAtomicUnit=on
  If Action Subsystem4 : Subsystem  TreatAsAtomicUnit=on
  If Action Subsystem5 : Subsystem  TreatAsAtomicUnit=on
  If1 : If  IfExpression=u1 < 30  ElseIfExpressions=u1 > 70
  Merge : Merge
  Merge1 : Merge  Inputs=3
  Random Integer Generator : commrandsrc3/Random Integer Generator  SetSize=10  SeedSource=Auto  Seed=0  SampleTime=1  SamplesPerFrame=1  OutputDataType=double  SimulateUsing=Interpreted execution
  Random Integer Generator1 : commrandsrc3/Random Integer Generator  SetSize=100  SeedSource=Auto  Seed=0  SampleTime=1  SamplesPerFrame=1  OutputDataType=double  SimulateUsing=Interpreted execution
  Random Integer Generator2 : commrandsrc3/Random Integer Generator  SetSize=100  SeedSource=Auto  Seed=0  SampleTime=1  SamplesPerFrame=1  OutputDataType=double  SimulateUsing=Interpreted execution
  Random Integer Generator3 : commrandsrc3/Random Integer Generator  SetSize=10  SeedSource=Auto  Seed=0  SampleTime=1  SamplesPerFrame=1  OutputDataType=double  SimulateUsing=Interpreted execution
  Random Integer Generator4 : commrandsrc3/Random Integer Generator  SetSize=10  SeedSource=Auto  Seed=0  SampleTime=1  SamplesPerFrame=1  OutputDataType=double  SimulateUsing=Interpreted execution
  Scope{,1..6} (7 alike) : Scope
  light : Switch  Criteria=u2 > Threshold
  light1 : Switch  Criteria=u2 > Threshold
  light2 : Switch  Criteria=u2 > Threshold
  wires:
  If Action Subsystem/1(Out1) -> Merge/1
  If/2 -> If Action Subsystem1/Action
  If/1 -> If Action Subsystem/Action
  If Action Subsystem1/1(Out1) -> Merge/2
  In1/1 -> Add/1
  Merge/1 -> Delay/1
  Add/1 -> Scope1/1, If/1
  Delay/1 -> Add/2
  If Action Subsystem4/1(Out1) -> Merge1/2
  If Action Subsystem5/1(Out1) -> Merge1/3
  If Action Subsystem3/1(Out1) -> Merge1/1
  Merge1/1 -> Delay1/1
  In2/1 -> Add1/1
  If1/3 -> If Action Subsystem5/Action
  If1/1 -> If Action Subsystem3/Action
  If1/2 -> If Action Subsystem4/Action
  Add1/1 -> Scope2/1, If1/1
  Delay1/1 -> Add1/2
  Random Integer Generator/1 -> light/2
  Constant/1 -> light/1
  Constant1/1 -> light/3
  light/1 -> Scope/1
  Constant2/1 -> Fire Alarm/1
  Constant3/1 -> Fire Alarm/3
  Random Integer Generator1/1 -> Fire Alarm/2
  Fire Alarm/1 -> Scope3/1
  Random Integer Generator2/1 -> Fire Alarm1/2
  Constant5/1 -> Fire Alarm1/3
  Fire Alarm1/1 -> Scope4/1
  Constant4/1 -> Fire Alarm1/1
  Constant6/1 -> light1/1
  Constant7/1 -> light1/3
  Random Integer Generator3/1 -> light1/2
  light1/1 -> Scope5/1
  Random Integer Generator4/1 -> light2/2
  light2/1 -> Scope6/1
  Constant8/1 -> light2/1
  Constant9/1 -> light2/3

== system smartHome6/corridor/If Action Subsystem ==
  Action Port : ActionPort  ActionType=then
  Constant : Constant  Value=10
  Out1 : Outport
  wires:
  Constant/1 -> Out1/1

== system smartHome6/corridor/If Action Subsystem1 ==
  Action Port : ActionPort  ActionType=elseif
  Constant : Constant  Value=-10
  Out1 : Outport
  wires:
  Constant/1 -> Out1/1

== system smartHome6/corridor/If Action Subsystem2 ==
  Action Port : ActionPort  ActionType=else
  Constant : Constant  Value=0
  Out1 : Outport
  wires:
  Constant/1 -> Out1/1

== system smartHome6/corridor/If Action Subsystem3 ==
  Action Port : ActionPort  ActionType=then
  Constant : Constant  Value=20
  Out1 : Outport
  wires:
  Constant/1 -> Out1/1

== system smartHome6/corridor/If Action Subsystem4 ==
  Action Port : ActionPort  ActionType=elseif
  Constant : Constant  Value=-10
  Out1 : Outport
  wires:
  Constant/1 -> Out1/1

== system smartHome6/corridor/If Action Subsystem5 ==
  Action Port : ActionPort  ActionType=else
  Constant : Constant  Value=0
  Out1 : Outport
  wires:
  Constant/1 -> Out1/1

== system smartHome6/corridor1/If Action Subsystem ==
  Action Port : ActionPort  ActionType=then
  Constant : Constant  Value=10
  Out1 : Outport
  wires:
  Constant/1 -> Out1/1

== system smartHome6/corridor1/If Action Subsystem1 ==
  Action Port : ActionPort  ActionType=elseif
  Constant : Constant  Value=-10
  Out1 : Outport
  wires:
  Constant/1 -> Out1/1

== system smartHome6/corridor1/If Action Subsystem2 ==
  Action Port : ActionPort  ActionType=else
  Constant : Constant  Value=0
  Out1 : Outport
  wires:
  Constant/1 -> Out1/1

== system smartHome6/corridor1/If Action Subsystem3 ==
  Action Port : ActionPort  ActionType=then
  Constant : Constant  Value=20
  Out1 : Outport
  wires:
  Constant/1 -> Out1/1

== system smartHome6/corridor1/If Action Subsystem4 ==
  Action Port : ActionPort  ActionType=elseif
  Constant : Constant  Value=-10
  Out1 : Outport
  wires:
  Constant/1 -> Out1/1

== system smartHome6/corridor1/If Action Subsystem5 ==
  Action Port : ActionPort  ActionType=else
  Constant : Constant  Value=0
  Out1 : Outport
  wires:
  Constant/1 -> Out1/1

== system smartHome6/room 1  testing 2/If Action Subsystem ==
  Action Port : ActionPort  ActionType=then
  Constant : Constant  Value=10
  Out1 : Outport
  wires:
  Constant/1 -> Out1/1

== system smartHome6/room 1  testing 2/If Action Subsystem1 ==
  Action Port : ActionPort  ActionType=elseif
  Constant : Constant  Value=-10
  Out1 : Outport
  wires:
  Constant/1 -> Out1/1

== system smartHome6/room 1  testing 2/If Action Subsystem10 ==
  Action Port : ActionPort  ActionType=elseif
  Constant : Constant  Value=-10
  Out1 : Outport
  wires:
  Constant/1 -> Out1/1

== system smartHome6/room 1  testing 2/If Action Subsystem11 ==
  Action Port : ActionPort  ActionType=else
  Constant : Constant  Value=0
  Out1 : Outport
  wires:
  Constant/1 -> Out1/1

== system smartHome6/room 1  testing 2/If Action Subsystem12 ==
  Action Port : ActionPort  ActionType=then
  Constant : Constant  Value=100
  Out1 : Outport
  wires:
  Constant/1 -> Out1/1

== system smartHome6/room 1  testing 2/If Action Subsystem13 ==
  Action Port : ActionPort  ActionType=elseif
  Constant : Constant  Value=-150
  Out1 : Outport
  wires:
  Constant/1 -> Out1/1

== system smartHome6/room 1  testing 2/If Action Subsystem14 ==
  Action Port : ActionPort  ActionType=else
  Constant : Constant  Value=0
  Out1 : Outport
  wires:
  Constant/1 -> Out1/1

== system smartHome6/room 1  testing 2/If Action Subsystem15 ==
  Action Port : ActionPort  ActionType=then
  Constant : Constant  Value=150
  Out1 : Outport
  wires:
  Constant/1 -> Out1/1

== system smartHome6/room 1  testing 2/If Action Subsystem16 ==
  Action Port : ActionPort  ActionType=else
  Constant : Constant  Value=0
  Out1 : Outport
  wires:
  Constant/1 -> Out1/1

== system smartHome6/room 1  testing 2/If Action Subsystem17 ==
  Action Port : ActionPort  ActionType=elseif
  Constant : Constant  Value=-10
  Out1 : Outport
  wires:
  Constant/1 -> Out1/1

== system smartHome6/room 1  testing 2/If Action Subsystem18 ==
  Action Port : ActionPort  ActionType=else
  Constant : Constant  Value=0
  Out1 : Outport
  wires:
  Constant/1 -> Out1/1

== system smartHome6/room 1  testing 2/If Action Subsystem19 ==
  Action Port : ActionPort  ActionType=then
  Constant : Constant  Value=10
  Out1 : Outport
  wires:
  Constant/1 -> Out1/1

== system smartHome6/room 1  testing 2/If Action Subsystem2 ==
  Action Port : ActionPort  ActionType=then
  Constant : Constant
  Out1 : Outport
  wires:
  Constant/1 -> Out1/1

== system smartHome6/room 1  testing 2/If Action Subsystem3 ==
  Action Port : ActionPort  ActionType=then
  Constant : Constant  Value=20
  Out1 : Outport
  wires:
  Constant/1 -> Out1/1

== system smartHome6/room 1  testing 2/If Action Subsystem4 ==
  Action Port : ActionPort  ActionType=elseif
  Constant : Constant  Value=-10
  Out1 : Outport
  wires:
  Constant/1 -> Out1/1

== system smartHome6/room 1  testing 2/If Action Subsystem5 ==
  Action Port : ActionPort  ActionType=else
  Constant : Constant  Value=0
  Out1 : Outport
  wires:
  Constant/1 -> Out1/1

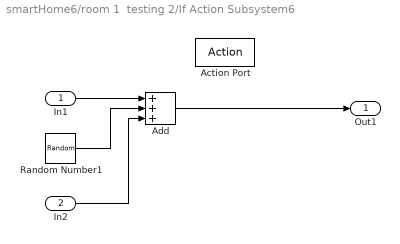
== system smartHome6/room 1  testing 2/If Action Subsystem6 ==
  In1 : Inport
  In2 : Inport  Port=2
  Action Port : ActionPort  ActionType=then
  Add : Sum  Inputs=+++
  Random Number1 : RandomNumber  Mean=10  Variance=3  SampleTime=1.0
  Out1 : Outport
  wires:
  In1/1 -> Add/1
  Add/1 -> Out1/1
  Random Number1/1 -> Add/2
  In2/1 -> Add/3

== system smartHome6/room 1  testing 2/If Action Subsystem7 ==
  Action Port : ActionPort  ActionType=else
  Constant : Constant  Value=0
  Out1 : Outport
  wires:
  Constant/1 -> Out1/1

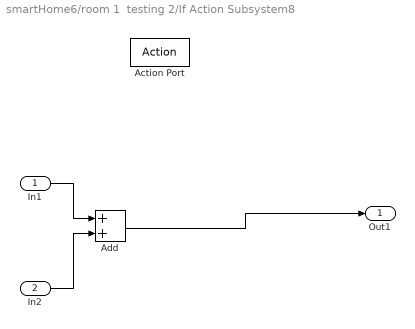
== system smartHome6/room 1  testing 2/If Action Subsystem8 ==
  In1 : Inport
  In2 : Inport  Port=2
  Action Port : ActionPort  ActionType=else
  Add : Sum
  Out1 : Outport
  wires:
  In2/1 -> Add/2
  In1/1 -> Add/1
  Add/1 -> Out1/1

== system smartHome6/room 1  testing 2/If Action Subsystem9 ==
  Action Port : ActionPort  ActionType=then
  Constant : Constant  Value=10
  Out1 : Outport
  wires:
  Constant/1 -> Out1/1

== system smartHome6/room 1 testing /If Action Subsystem ==
  Action Port : ActionPort  ActionType=then
  Constant : Constant  Value=10
  Out1 : Outport
  wires:
  Constant/1 -> Out1/1

== system smartHome6/room 1 testing /If Action Subsystem1 ==
  Action Port : ActionPort  ActionType=elseif
  Constant : Constant  Value=-10
  Out1 : Outport
  wires:
  Constant/1 -> Out1/1

== system smartHome6/room 1 testing /If Action Subsystem2 ==
  Action Port : ActionPort  ActionType=then
  Constant : Constant
  Out1 : Outport
  wires:
  Constant/1 -> Out1/1

== system smartHome6/room 1 testing /If Action Subsystem3 ==
  Action Port : ActionPort  ActionType=then
  Constant : Constant  Value=20
  Out1 : Outport
  wires:
  Constant/1 -> Out1/1

== system smartHome6/room 1 testing /If Action Subsystem4 ==
  Action Port : ActionPort  ActionType=elseif
  Constant : Constant  Value=-10
  Out1 : Outport
  wires:
  Constant/1 -> Out1/1

== system smartHome6/room 1 testing /If Action Subsystem5 ==
  Action Port : ActionPort  ActionType=else
  Constant : Constant  Value=0
  Out1 : Outport
  wires:
  Constant/1 -> Out1/1

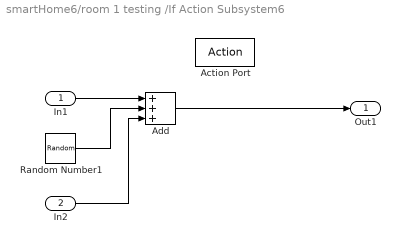
== system smartHome6/room 1 testing /If Action Subsystem6 ==
  In1 : Inport
  In2 : Inport  Port=2
  Action Port : ActionPort  ActionType=then
  Add : Sum  Inputs=+++
  Random Number1 : RandomNumber  Mean=3  Variance=3  SampleTime=1.0
  Out1 : Outport
  wires:
  In1/1 -> Add/1
  Add/1 -> Out1/1
  Random Number1/1 -> Add/2
  In2/1 -> Add/3

== system smartHome6/room 1 testing /If Action Subsystem7 ==
  Action Port : ActionPort  ActionType=else
  Constant : Constant  Value=0
  Out1 : Outport
  wires:
  Constant/1 -> Out1/1

== system smartHome6/room 1 testing /If Action Subsystem8 ==
  In1 : Inport
  In2 : Inport  Port=2
  Action Port : ActionPort  ActionType=else
  Add : Sum
  Out1 : Outport
  wires:
  In2/1 -> Add/2
  In1/1 -> Add/1
  Add/1 -> Out1/1

== system smartHome6/room 2/If Action Subsystem ==
  Action Port : ActionPort  ActionType=then
  Constant : Constant  Value=10
  Out1 : Outport
  wires:
  Constant/1 -> Out1/1

== system smartHome6/room 2/If Action Subsystem1 ==
  Action Port : ActionPort  ActionType=elseif
  Constant : Constant  Value=-10
  Out1 : Outport
  wires:
  Constant/1 -> Out1/1

== system smartHome6/room 2/If Action Subsystem2 ==
  Action Port : ActionPort  ActionType=else
  Constant : Constant  Value=0
  Out1 : Outport
  wires:
  Constant/1 -> Out1/1

== system smartHome6/room 2/If Action Subsystem3 ==
  Action Port : ActionPort  ActionType=then
  Constant : Constant  Value=20
  Out1 : Outport
  wires:
  Constant/1 -> Out1/1

== system smartHome6/room 2/If Action Subsystem4 ==
  Action Port : ActionPort  ActionType=elseif
  Constant : Constant  Value=-10
  Out1 : Outport
  wires:
  Constant/1 -> Out1/1

== system smartHome6/room 2/If Action Subsystem5 ==
  Action Port : ActionPort  ActionType=else
  Constant : Constant  Value=0
  Out1 : Outport
  wires:
  Constant/1 -> Out1/1

== system smartHome6/room 2 testing /If Action Subsystem ==
  Action Port : ActionPort  ActionType=then
  Constant : Constant  Value=10
  Out1 : Outport
  wires:
  Constant/1 -> Out1/1

== system smartHome6/room 2 testing /If Action Subsystem1 ==
  Action Port : ActionPort  ActionType=elseif
  Constant : Constant  Value=-10
  Out1 : Outport
  wires:
  Constant/1 -> Out1/1

== system smartHome6/room 2 testing /If Action Subsystem2 ==
  Action Port : ActionPort  ActionType=then
  Constant : Constant
  Out1 : Outport
  wires:
  Constant/1 -> Out1/1

== system smartHome6/room 2 testing /If Action Subsystem3 ==
  Action Port : ActionPort  ActionType=then
  Constant : Constant  Value=20
  Out1 : Outport
  wires:
  Constant/1 -> Out1/1

== system smartHome6/room 2 testing /If Action Subsystem4 ==
  Action Port : ActionPort  ActionType=elseif
  Constant : Constant  Value=-10
  Out1 : Outport
  wires:
  Constant/1 -> Out1/1

== system smartHome6/room 2 testing /If Action Subsystem5 ==
  Action Port : ActionPort  ActionType=else
  Constant : Constant  Value=0
  Out1 : Outport
  wires:
  Constant/1 -> Out1/1

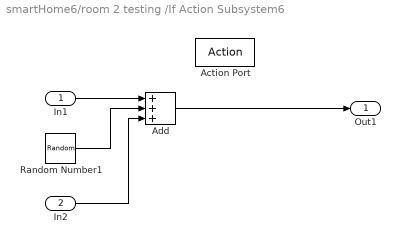
== system smartHome6/room 2 testing /If Action Subsystem6 ==
  In1 : Inport
  In2 : Inport  Port=2
  Action Port : ActionPort  ActionType=then
  Add : Sum  Inputs=+++
  Random Number1 : RandomNumber  Mean=3  Variance=3  SampleTime=1.0
  Out1 : Outport
  wires:
  In1/1 -> Add/1
  Add/1 -> Out1/1
  Random Number1/1 -> Add/2
  In2/1 -> Add/3

== system smartHome6/room 2 testing /If Action Subsystem7 ==
  Action Port : ActionPort  ActionType=else
  Constant : Constant  Value=0
  Out1 : Outport
  wires:
  Constant/1 -> Out1/1

== system smartHome6/room 2 testing /If Action Subsystem8 ==
  In1 : Inport
  In2 : Inport  Port=2
  Action Port : ActionPort  ActionType=else
  Add : Sum
  Out1 : Outport
  wires:
  In2/1 -> Add/2
  In1/1 -> Add/1
  Add/1 -> Out1/1

== system smartHome6/room1/If Action Subsystem ==
  Action Port : ActionPort  ActionType=then
  Constant : Constant  Value=10
  Out1 : Outport
  wires:
  Constant/1 -> Out1/1

== system smartHome6/room1/If Action Subsystem1 ==
  Action Port : ActionPort  ActionType=elseif
  Constant : Constant  Value=-10
  Out1 : Outport
  wires:
  Constant/1 -> Out1/1

== system smartHome6/room1/If Action Subsystem3 ==
  Action Port : ActionPort  ActionType=then
  Constant : Constant  Value=20
  Out1 : Outport
  wires:
  Constant/1 -> Out1/1

== system smartHome6/room1/If Action Subsystem4 ==
  Action Port : ActionPort  ActionType=elseif
  Constant : Constant  Value=-10
  Out1 : Outport
  wires:
  Constant/1 -> Out1/1

== system smartHome6/room1/If Action Subsystem5 ==
  Action Port : ActionPort  ActionType=else
  Constant : Constant  Value=0
  Out1 : Outport
  wires:
  Constant/1 -> Out1/1
